simulink model "airgk"  (Simulink 3.00)
settings: Solver=ode45  StartTime=0  StopTime=Inf  RelTol=1e-3
libraries: simulink3 x21, airlib x1
(part 2 of 2)

== system airgk/uy-Control/uDynInv/Inertia Products ==
  w : Inport  Port=1  PortWidth=-1  SampleTime=-1  DataType=auto
      settings: SignalType=auto
  wd : Inport  Port=2  PortWidth=-1  SampleTime=-1  DataType=auto
      settings: SignalType=auto
  3x1mult : Subsystem
      mask Type: 3x1 Matrix Multiplication
      mask Description:
      | Input 1   : elements of matrix X (3 by 3)
      |   Input 2   : elements of matrix Y (3 by 1)
      |   Output   : elements of matrix X*Y (3 by 1)
      mask Help:
      | <p>
      | Elements of input and output matrices are taken columnwise.
      | </p>
      mask Display: disp('Z=X*Y')
  3x1mult1 : Subsystem
      mask Type: 3x1 Matrix Multiplication
      mask Description:
      | Input 1   : elements of matrix X (3 by 3)
      |   Input 2   : elements of matrix Y (3 by 1)
      |   Output   : elements of matrix X*Y (3 by 1)
      mask Help:
      | <p>
      | Elements of input and output matrices are taken columnwise.
      | </p>
      mask Display: disp('Z=X*Y')
  3x1mult2 : Subsystem
      mask Type: 3x1 Matrix Multiplication
      mask Description:
      | Input 1   : elements of matrix X (3 by 3)
      |   Input 2   : elements of matrix Y (3 by 1)
      |   Output   : elements of matrix X*Y (3 by 1)
      mask Help:
      | <p>
      | Elements of input and output matrices are taken columnwise.
      | </p>
      mask Display: disp('Z=X*Y')
  Inertia Matrix : Constant  Value=[GM1(4) -GM1(7) -GM1(8) -GM1(7) GM1(5) -GM1(9) -GM1(8) -GM1(9) GM1(6)]
  Sum : Sum  Inputs=|++  SaturateOnIntegerOverflow=on
  w2W : Subsystem
      mask Display: disp('S')
  W*J*w+J*wt : Outport  Port=1
  wires:
  w2W/1(Out1) -> 3x1mult2/1(X)
  3x1mult1/1(Z) -> 3x1mult2/2(Y)
  w/1 -> 3x1mult1/2(Y), w2W/1(In1)
  3x1mult/1(Z) -> Sum/1
  3x1mult2/1(Z) -> Sum/2
  Sum/1 -> W*J*w+J*wt/1
  wd/1 -> 3x1mult/2(Y)
  Inertia Matrix/1 -> 3x1mult/1(X), 3x1mult1/1(X)

== system airgk/uy-Control/uDynInv/Inv Rot ==
  w : Inport  Port=1  PortWidth=-1  SampleTime=-1  DataType=auto
      settings: SignalType=auto
  ftp : Inport  Port=2  PortWidth=-1  SampleTime=-1  DataType=auto
      settings: SignalType=auto
  add : Inport  Port=3  PortWidth=-1  SampleTime=-1  DataType=auto
      settings: SignalType=auto
  M : Subsystem
      mask Type: Simulink Matrix Library Block
      mask Description:
      | Roll, Pitch and Yaw derivatives to Omega :
      |   Input 1 : Roll, Pitch and Yaw angles (phi,theta,psi)
      |   Input 2 : Roll, Pitch and Yaw derivatives
      |   Output : Omega (p,q,r)
      mask Help:
      | <p>
      | Roll, Pitch and Yaw angles express the orientation
      | of the Body frame with respect to the Earth frame.
      | </p>
      | <p>
      | To use this block you should have the smxl library in your path.
      | </p>
  Sum1 : Sum  Inputs=+++  SaturateOnIntegerOverflow=on
  dM/df : Subsystem
  dM/dt : Subsystem
  pqr2ftpdot : Subsystem
      mask Type: Simulink Matrix Library Block
      mask Description:
      | Omega to Roll, Pitch and Yaw derivatives :
      |   Input 1 : Roll, Pitch and Yaw angles (phi,theta,psi)
      |   Input 2 : Omega (p,q,r)
      |   Output : Roll, Pitch and Yaw derivatives
      mask Help:
      | <p>
      | Roll, Pitch and Yaw angles express the orientation
      | of the Body frame with respect to the Earth frame.
      | </p>
      | <p>
      | To use this block you should have the smxl library in your path.
      | </p>
  wd : Outport  Port=1
  wires:
  add/1 -> M/2(ftpdot)
  ftp/1 -> pqr2ftpdot/1(ftp), M/1(ftp), dM/df/1(ftp), dM/dt/1(ftp)
  w/1 -> pqr2ftpdot/2(pqr)
  pqr2ftpdot/1(ftpdot) -> dM/dt/2(ftpd), dM/df/2(ftpd)
  M/1(pqr) -> Sum1/3
  dM/dt/1(Tt) -> Sum1/1
  dM/df/1(Tf) -> Sum1/2
  Sum1/1 -> wd/1

== system airgk/uy-Control/uDynInv/ad1 ==
  x : Inport  Port=1  PortWidth=-1  SampleTime=-1  DataType=auto
      settings: SignalType=auto
  yatm : Inport  Port=2  PortWidth=-1  SampleTime=-1  DataType=auto
      settings: SignalType=auto
  0 : Subsystem
      settings: OpenFcn=fdchelp airdata1
      mask Display: disp('AIRDATA1\nM.O. Rauw, October 1997')
  M : Fcn  Expr=u[2]/u[1]
  Mux : Mux  Inputs=[1 12]
      settings: DisplayOption=none
  Mux1 : Mux  Inputs=[12 5]
      settings: DisplayOption=none
  Mux2 : Mux  Inputs=3
      settings: DisplayOption=none
  a : Fcn  Expr=sqrt(401.8743*u[3])
  qdyn : Fcn  Expr=0.5*u[13]*u[1]^2
  yad1 : Outport  Port=1
  wires:
  yatm/1 -> Mux1/2, a/1
  x/1 -> Mux1/1, Mux/2
  Mux/1 -> M/1
  Mux1/1 -> qdyn/1
  M/1 -> Mux2/2
  a/1 -> Mux2/1, Mux/1
  qdyn/1 -> Mux2/3
  Mux2/1 -> yad1/1

== system airgk/uy-Control/uDynInv/atm ==
  x : Inport  Port=1  PortWidth=-1  SampleTime=-1  DataType=auto
      settings: SignalType=auto
  0 : Subsystem
      settings: OpenFcn=fdchelp atmosph
      mask Display: disp('ATMOSPH\nM.O. Rauw, October 1997')
  Mux : Mux  Inputs=2
      settings: DisplayOption=none
  Mux1 : Mux  Inputs=[2 1]
      settings: DisplayOption=none
  Mux2 : Mux  Inputs=5
      settings: DisplayOption=none
  T : Fcn  Expr=288.15 - 0.0065*u[12]
  g : Fcn  Expr=9.80665*(6371020/(6371020+u[12]))^2
  mu : Fcn  Expr=(1.458*10^(-6)*u[2]^1.5)/(u[2]+110.4)
  ps : Fcn  Expr=101325*(u[2]/288.15)^(u[1]/1.86584)
  rho : Fcn  Expr=u[3]/(287.053*u[2])
  yatm : Outport  Port=1
  wires:
  mu/1 -> Mux2/4
  Mux2/1 -> yatm/1
  Mux1/1 -> rho/1
  rho/1 -> Mux2/1
  g/1 -> Mux2/5, Mux/1
  T/1 -> Mux2/3, Mux/2
  ps/1 -> Mux2/2, Mux1/2
  Mux/1 -> ps/1, mu/1, Mux1/1
  x/1 -> g/1, T/1

== system airgk/uy-Control/uDynInv/dl ==
  x : Inport  Port=1  PortWidth=-1  SampleTime=-1  DataType=auto
      settings: SignalType=auto
  0 : Subsystem
      settings: OpenFcn=fdchelp dimless
      mask Display: disp('DIMLESS\nM.O. Rauw, October 1997')
  Mux : Mux  Inputs=3
      settings: DisplayOption=none
  pb/2V : Fcn  Expr=0.5 * u[4] * b / u[1]
  qc/2V : Fcn  Expr=0.5* u[5] * cbar / u[1]
  rb/2V : Fcn  Expr=0.5 * u[6] * b / u[1]
  ydl : Outport  Port=1
  wires:
  pb/2V/1 -> Mux/1
  qc/2V/1 -> Mux/2
  rb/2V/1 -> Mux/3
  Mux/1 -> ydl/1
  x/1 -> qc/2V/1, rb/2V/1, pb/2V/1

== system airgk/uy-Control/uDynInv/inv AM_CM ==
  In1 : Inport  Port=1  PortWidth=-1  SampleTime=-1  DataType=auto
      settings: SignalType=auto
  Matrix Gain : StateSpace  A=[]  B=[]  C=[]  D=M  X0=0
  Out1 : Outport  Port=1
  wires:
  In1/1 -> Matrix Gain/1
  Matrix Gain/1 -> Out1/1

== system airgk/uy-Control/4CmdsuKinInv/Exact Turn Coordination/Derivative ==
  x : Inport  Orientation=left  Port=1  PortWidth=-1  SampleTime=-1  DataType=auto
      settings: SignalType=auto
  Product2 : Product  Orientation=left  Inputs=/*  SaturateOnIntegerOverflow=on
  Sum4 : Sum  Orientation=left  Inputs=|+-  SaturateOnIntegerOverflow=on
  Unit Delay1 : UnitDelay  Orientation=left  X0=x0  SampleTime=T
  Zero-Order Hold1 : ZeroOrderHold  Orientation=left  SampleTime=T
  m : Constant  Orientation=left  Value=T
  xdot : Outport  Orientation=left  Port=1
  wires:
  Sum4/1 -> Product2/2
  Unit Delay1/1 -> Sum4/2
  Zero-Order Hold1/1 -> Sum4/1, Unit Delay1/1
  m/1 -> Product2/1
  Product2/1 -> xdot/1
  x/1 -> Zero-Order Hold1/1

== system airgk/uy-Control/4CmdsuKinInv/a2c  xy/Derivative ==
  x : Inport  Orientation=left  Port=1  PortWidth=-1  SampleTime=-1  DataType=auto
      settings: SignalType=auto
  Product2 : Product  Orientation=left  Inputs=/*  SaturateOnIntegerOverflow=on
  Sum4 : Sum  Orientation=left  Inputs=|+-  SaturateOnIntegerOverflow=on
  Unit Delay1 : UnitDelay  Orientation=left  X0=0  SampleTime=-1
  Zero-Order Hold1 : ZeroOrderHold  Orientation=left  SampleTime=T
  m : Constant  Orientation=left  Value=T
  xdot : Outport  Orientation=left  Port=1
  wires:
  x/1 -> Zero-Order Hold1/1
  Product2/1 -> xdot/1
  m/1 -> Product2/1
  Zero-Order Hold1/1 -> Unit Delay1/1, Sum4/1
  Unit Delay1/1 -> Sum4/2
  Sum4/1 -> Product2/2

== system airgk/uy-Control/4CmdsuKinInv/a2c xz/Derivative ==
  x : Inport  Orientation=left  Port=1  PortWidth=-1  SampleTime=-1  DataType=auto
      settings: SignalType=auto
  Product2 : Product  Orientation=left  Inputs=/*  SaturateOnIntegerOverflow=on
  Sum4 : Sum  Orientation=left  Inputs=|+-  SaturateOnIntegerOverflow=on
  Unit Delay1 : UnitDelay  Orientation=left  X0=0  SampleTime=-1
  Zero-Order Hold1 : ZeroOrderHold  Orientation=left  SampleTime=T
  m : Constant  Orientation=left  Value=T
  xdot : Outport  Orientation=left  Port=1
  wires:
  Sum4/1 -> Product2/2
  Unit Delay1/1 -> Sum4/2
  Zero-Order Hold1/1 -> Sum4/1, Unit Delay1/1
  m/1 -> Product2/1
  Product2/1 -> xdot/1
  x/1 -> Zero-Order Hold1/1

== system airgk/uy-Control/Vcmd Generator/xyHdot/3x1 ==
  X : Inport  Port=1  PortWidth=-1  SampleTime=-1  DataType=auto
      settings: SignalType=auto
  Y : Inport  Port=2  PortWidth=-1  SampleTime=-1  DataType=auto
      settings: SignalType=auto
  Dot Product1 : Subsystem  mask(Dot Product){}
      mask help:
      | Inner (dot) product.
      | y = sum(conj(u1).*u2). The operand u1 corresponds to the top (or left) input port.
      mask init:
      | t=(0:.1:2*pi)';
      | x=cos(t);
      | y=sin(t);
      | r=0.05;
      mask Help: Computes the inner (dot) product of the inputs: sum(u1.*u2).  The inputs are vectors of the same length. Output is a scalar.
      mask Display: patch([x*r+0.5],[y*r+0.5])
  Dot Product2 : Subsystem  mask(Dot Product){}
      mask help:
      | Inner (dot) product.
      | y = sum(conj(u1).*u2). The operand u1 corresponds to the top (or left) input port.
      mask init:
      | t=(0:.1:2*pi)';
      | x=cos(t);
      | y=sin(t);
      | r=0.05;
      mask Help: Computes the inner (dot) product of the inputs: sum(u1.*u2).  The inputs are vectors of the same length. Output is a scalar.
      mask Display: patch([x*r+0.5],[y*r+0.5])
  Dot Product9 : Subsystem  mask(Dot Product){}
      mask help:
      | Inner (dot) product.
      | y = sum(conj(u1).*u2). The operand u1 corresponds to the top (or left) input port.
      mask init:
      | t=(0:.1:2*pi)';
      | x=cos(t);
      | y=sin(t);
      | r=0.05;
      mask Help: Computes the inner (dot) product of the inputs: sum(u1.*u2).  The inputs are vectors of the same length. Output is a scalar.
      mask Display: patch([x*r+0.5],[y*r+0.5])
  Gain : Gain  Gain=-1  SaturateOnIntegerOverflow=off
  Mux : Mux  Inputs=3
  Selector : Selector  Elements=[1:3]  InputPortWidth=9
  Selector1 : Selector  Elements=[4:6]  InputPortWidth=9
  Selector2 : Selector  Elements=[7:9]  InputPortWidth=9
  Z : Outport  Port=1
  wires:
  Mux/1 -> Z/1
  Selector2/1 -> Dot Product2/1(In1)
  Selector1/1 -> Dot Product1/1(In1)
  Y/1 -> Dot Product9/2(In2), Dot Product1/2(In2), Dot Product2/2(In2)
  Dot Product2/1(Out1) -> Gain/1
  Dot Product1/1(Out1) -> Mux/2
  Dot Product9/1(Out1) -> Mux/1
  Selector/1 -> Dot Product9/1(In1)
  X/1 -> Selector2/1, Selector1/1, Selector/1
  Gain/1 -> Mux/3

== system airgk/uy-Control/Vcmd Generator/xyHdot/SinCos ==
  theta : Inport  Port=1  PortWidth=-1  SampleTime=-1  DataType=auto
      settings: SignalType=auto
  cosine : Trigonometry  Operator=cos  OutputSignalType=auto
  sine : Trigonometry  Operator=sin  OutputSignalType=auto
  sin(theta) : Outport  Port=1
  cos(theta) : Outport  Port=2
  wires:
  cosine/1 -> cos(theta)/1
  sine/1 -> sin(theta)/1
  theta/1 -> cosine/1, sine/1

== system airgk/uy-Control/uDynInv/ u term/uvw ==
  x : Inport  Port=1  PortWidth=-1  SampleTime=-1  DataType=auto
      settings: SignalType=auto
  Mux : Mux  Inputs=3
      settings: DisplayOption=none
  u : Fcn  Expr=u[1]*cos(u[2])*cos(u[3])
  v : Fcn  Expr=u[1]*sin(u[3])
  w : Fcn  Expr=u[1]*sin(u[2])*cos(u[3])
  ybvel : Outport  Port=1
  wires:
  Mux/1 -> ybvel/1
  w/1 -> Mux/3
  v/1 -> Mux/2
  u/1 -> Mux/1
  x/1 -> v/1, w/1, u/1

== system airgk/uy-Control/uDynInv/Inertia Products/3x1mult ==
  X : Inport  Port=1  PortWidth=-1  SampleTime=-1  DataType=auto
      settings: SignalType=auto
  Y : Inport  Port=2  PortWidth=-1  SampleTime=-1  DataType=auto
      settings: SignalType=auto
  Dot Product : simulink3/Math/Dot Product
  Dot Product1 : simulink3/Math/Dot Product
  Dot Product2 : simulink3/Math/Dot Product
  Mux : Mux  Inputs=3
  Selector : Selector  Elements=[0 3 6]+1  InputPortWidth=9
  Selector1 : Selector  Elements=[0 3 6]+2  InputPortWidth=9
  Selector2 : Selector  Elements=[0 3 6]+3  InputPortWidth=9
  Z : Outport  Port=1
  wires:
  Y/1 -> Dot Product/2, Dot Product1/2, Dot Product2/2
  Selector2/1 -> Dot Product2/1
  Selector1/1 -> Dot Product1/1
  Selector/1 -> Dot Product/1
  Mux/1 -> Z/1
  Dot Product2/1 -> Mux/3
  Dot Product1/1 -> Mux/2
  Dot Product/1 -> Mux/1
  X/1 -> Selector2/1, Selector1/1, Selector/1

== system airgk/uy-Control/uDynInv/Inertia Products/3x1mult1 ==
  X : Inport  Port=1  PortWidth=-1  SampleTime=-1  DataType=auto
      settings: SignalType=auto
  Y : Inport  Port=2  PortWidth=-1  SampleTime=-1  DataType=auto
      settings: SignalType=auto
  Dot Product : simulink3/Math/Dot Product
  Dot Product1 : simulink3/Math/Dot Product
  Dot Product2 : simulink3/Math/Dot Product
  Mux : Mux  Inputs=3
  Selector : Selector  Elements=[0 3 6]+1  InputPortWidth=9
  Selector1 : Selector  Elements=[0 3 6]+2  InputPortWidth=9
  Selector2 : Selector  Elements=[0 3 6]+3  InputPortWidth=9
  Z : Outport  Port=1
  wires:
  Y/1 -> Dot Product/2, Dot Product1/2, Dot Product2/2
  Selector2/1 -> Dot Product2/1
  Selector1/1 -> Dot Product1/1
  Selector/1 -> Dot Product/1
  Mux/1 -> Z/1
  Dot Product2/1 -> Mux/3
  Dot Product1/1 -> Mux/2
  Dot Product/1 -> Mux/1
  X/1 -> Selector2/1, Selector1/1, Selector/1

== system airgk/uy-Control/uDynInv/Inertia Products/3x1mult2 ==
  X : Inport  Port=1  PortWidth=-1  SampleTime=-1  DataType=auto
      settings: SignalType=auto
  Y : Inport  Port=2  PortWidth=-1  SampleTime=-1  DataType=auto
      settings: SignalType=auto
  Dot Product : simulink3/Math/Dot Product
  Dot Product1 : simulink3/Math/Dot Product
  Dot Product2 : simulink3/Math/Dot Product
  Mux : Mux  Inputs=3
  Selector : Selector  Elements=[0 3 6]+1  InputPortWidth=9
  Selector1 : Selector  Elements=[0 3 6]+2  InputPortWidth=9
  Selector2 : Selector  Elements=[0 3 6]+3  InputPortWidth=9
  Z : Outport  Port=1
  wires:
  Y/1 -> Dot Product/2, Dot Product1/2, Dot Product2/2
  Selector2/1 -> Dot Product2/1
  Selector1/1 -> Dot Product1/1
  Selector/1 -> Dot Product/1
  Mux/1 -> Z/1
  Dot Product2/1 -> Mux/3
  Dot Product1/1 -> Mux/2
  Dot Product/1 -> Mux/1
  X/1 -> Selector2/1, Selector1/1, Selector/1

== system airgk/uy-Control/uDynInv/Inertia Products/w2W ==
  In1 : Inport  Port=1  PortWidth=-1  SampleTime=-1  DataType=auto
      settings: SignalType=auto
  State Space : StateSpace  A=[]  B=[]  C=[]  D=[0 0 0;0 0 1;0 -1 0;0 0 -1;0 0 0;1 0 0;0 1 0;-1 0 0;0 0 0]  X0=0
  Out1 : Outport  Port=1
  wires:
  State Space/1 -> Out1/1
  In1/1 -> State Space/1

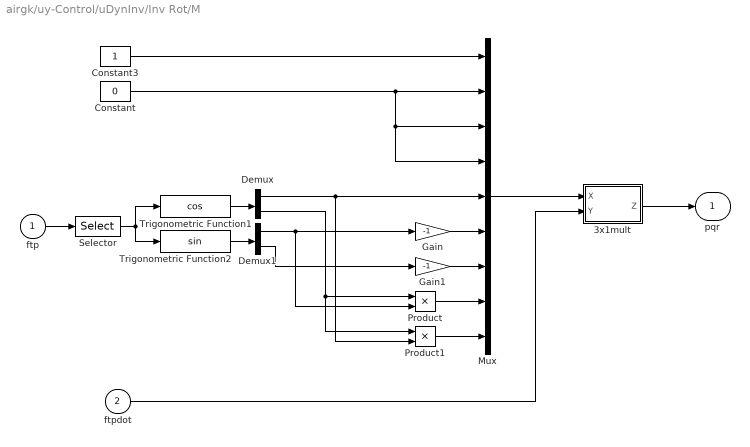
== system airgk/uy-Control/uDynInv/Inv Rot/M ==
  ftp : Inport  Port=1  PortWidth=-1  SampleTime=-1  DataType=auto
      settings: SignalType=auto
  ftpdot : Inport  Port=2  PortWidth=-1  SampleTime=-1  DataType=auto
      settings: SignalType=auto
  3x1mult : Subsystem
      mask Type: 3x1 Matrix Multiplication
      mask Description:
      | Input 1   : elements of matrix X (3 by 3)
      |   Input 2   : elements of matrix Y (3 by 1)
      |   Output   : elements of matrix X*Y (3 by 1)
      mask Help:
      | <p>
      | Elements of input and output matrices are taken columnwise.
      | </p>
      mask Display: disp('Z=X*Y')
  Constant : Constant  Value=0
  Constant3 : Constant  Value=1
  Demux : Demux  Outputs=2
  Demux1 : Demux  Outputs=2
  Gain : Gain  Gain=-1  SaturateOnIntegerOverflow=on
  Gain1 : Gain  Gain=-1  SaturateOnIntegerOverflow=on
  Mux : Mux  Inputs=9
  Product : Product  Inputs=2  SaturateOnIntegerOverflow=on
  Product1 : Product  Inputs=2  SaturateOnIntegerOverflow=on
  Selector : Selector  Elements=[1 2]  InputPortWidth=3
  Trigonometric Function1 : Trigonometry  Operator=cos  OutputSignalType=auto
  Trigonometric Function2 : Trigonometry  Operator=sin  OutputSignalType=auto
  pqr : Outport  Port=1
  wires:
  Constant3/1 -> Mux/1
  Constant/1 -> Mux/2, Mux/3, Mux/4
  Gain/1 -> Mux/6
  Gain1/1 -> Mux/7
  Trigonometric Function1/1 -> Demux/1
  Demux1/2 -> Gain1/1
  Product/1 -> Mux/8
  Product1/1 -> Mux/9
  Demux/2 -> Product/1, Product1/1
  Demux/1 -> Mux/5, Product1/2
  Selector/1 -> Trigonometric Function1/1, Trigonometric Function2/1
  ftpdot/1 -> 3x1mult/2(Y)
  Mux/1 -> 3x1mult/1(X)
  3x1mult/1(Z) -> pqr/1
  Trigonometric Function2/1 -> Demux1/1
  Demux1/1 -> Gain/1, Product/2
  ftp/1 -> Selector/1

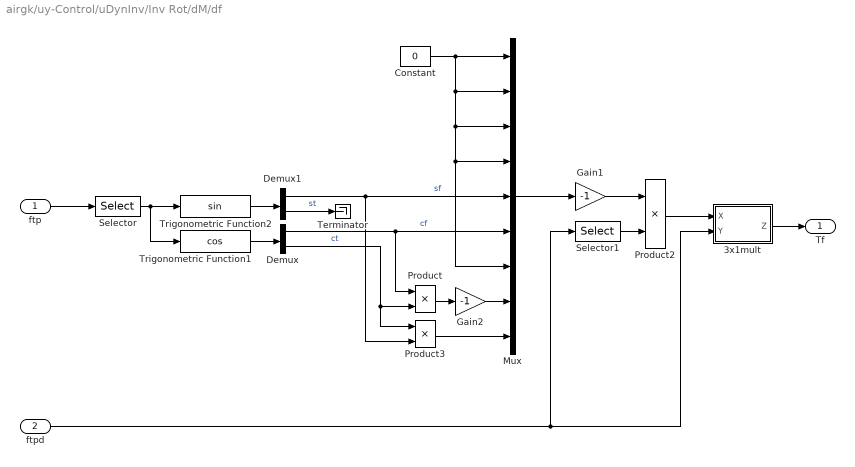
== system airgk/uy-Control/uDynInv/Inv Rot/dM/df ==
  ftp : Inport  Port=1  PortWidth=-1  SampleTime=-1  DataType=auto
      settings: SignalType=auto
  ftpd : Inport  Port=2  PortWidth=-1  SampleTime=-1  DataType=auto
      settings: SignalType=auto
  3x1mult : Subsystem
      mask Type: 3x1 Matrix Multiplication
      mask Description:
      | Input 1   : elements of matrix X (3 by 3)
      |   Input 2   : elements of matrix Y (3 by 1)
      |   Output   : elements of matrix X*Y (3 by 1)
      mask Help:
      | <p>
      | Elements of input and output matrices are taken columnwise.
      | </p>
      mask Display: disp('Z=X*Y')
  Constant : Constant  Value=0
  Demux : Demux  Outputs=2
  Demux1 : Demux  Outputs=2
  Gain1 : Gain  Gain=-1  SaturateOnIntegerOverflow=on
  Gain2 : Gain  Gain=-1  SaturateOnIntegerOverflow=on
  Mux : Mux  Inputs=9
  Product : Product  Inputs=2  SaturateOnIntegerOverflow=on
  Product2 : Product  Inputs=2  SaturateOnIntegerOverflow=on
  Product3 : Product  Inputs=2  SaturateOnIntegerOverflow=on
  Selector : Selector  Elements=[1 2]  InputPortWidth=3
  Selector1 : Selector  Elements=1  InputPortWidth=3
  Terminator : Terminator
  Trigonometric Function1 : Trigonometry  Operator=cos  OutputSignalType=auto
  Trigonometric Function2 : Trigonometry  Operator=sin  OutputSignalType=auto
  Tf : Outport  Port=1
  wires:
  3x1mult/1(Z) -> Tf/1
  Selector1/1 -> Product2/2
  Product2/1 -> 3x1mult/1(X)
  ftpd/1 -> Selector1/1, 3x1mult/2(Y)
  Gain1/1 -> Product2/1
  Mux/1 -> Gain1/1
  Constant/1 -> Mux/3, Mux/4, Mux/7, Mux/2, Mux/1
  ftp/1 -> Selector/1
  Trigonometric Function2/1 -> Demux1/1
  Selector/1 -> Trigonometric Function2/1, Trigonometric Function1/1
  Trigonometric Function1/1 -> Demux/1
  Demux1/1 -> Mux/5, Product3/2  "sf"
  Demux/1 -> Mux/6, Product/1  "cf"
  Product/1 -> Gain2/1
  Demux/2 -> Product/2, Product3/1  "ct"
  Product3/1 -> Mux/9
  Demux1/2 -> Terminator/1  "st"
  Gain2/1 -> Mux/8

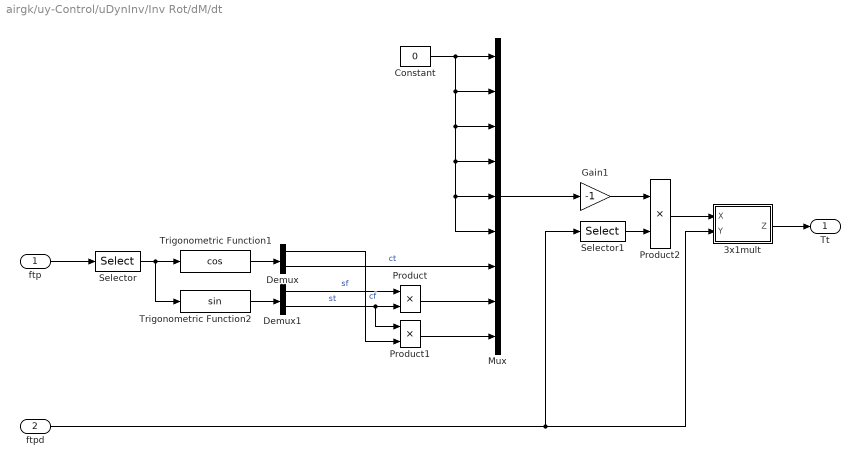
== system airgk/uy-Control/uDynInv/Inv Rot/dM/dt ==
  ftp : Inport  Port=1  PortWidth=-1  SampleTime=-1  DataType=auto
      settings: SignalType=auto
  ftpd : Inport  Port=2  PortWidth=-1  SampleTime=-1  DataType=auto
      settings: SignalType=auto
  3x1mult : Subsystem
      mask Type: 3x1 Matrix Multiplication
      mask Description:
      | Input 1   : elements of matrix X (3 by 3)
      |   Input 2   : elements of matrix Y (3 by 1)
      |   Output   : elements of matrix X*Y (3 by 1)
      mask Help:
      | <p>
      | Elements of input and output matrices are taken columnwise.
      | </p>
      mask Display: disp('Z=X*Y')
  Constant : Constant  Value=0
  Demux : Demux  Outputs=2
  Demux1 : Demux  Outputs=2
  Gain1 : Gain  Gain=-1  SaturateOnIntegerOverflow=on
  Mux : Mux  Inputs=9
  Product : Product  Inputs=2  SaturateOnIntegerOverflow=on
  Product1 : Product  Inputs=2  SaturateOnIntegerOverflow=on
  Product2 : Product  Inputs=2  SaturateOnIntegerOverflow=on
  Selector : Selector  Elements=[1 2]  InputPortWidth=3
  Selector1 : Selector  Elements=2  InputPortWidth=3
  Trigonometric Function1 : Trigonometry  Operator=cos  OutputSignalType=auto
  Trigonometric Function2 : Trigonometry  Operator=sin  OutputSignalType=auto
  Tt : Outport  Port=1
  wires:
  Trigonometric Function1/1 -> Demux/1
  Selector/1 -> Trigonometric Function2/1, Trigonometric Function1/1
  Trigonometric Function2/1 -> Demux1/1
  ftp/1 -> Selector/1
  Constant/1 -> Mux/1, Mux/2, Mux/3, Mux/4, Mux/5, Mux/6
  Demux/2 -> Mux/7  "ct"
  Product/1 -> Mux/8
  Product1/1 -> Mux/9
  Mux/1 -> Gain1/1
  Gain1/1 -> Product2/1
  Demux1/1 -> Product/1  "sf"
  Demux1/2 -> Product/2, Product1/1  "st"
  Demux/1 -> Product1/2  "cf"
  ftpd/1 -> 3x1mult/2(Y), Selector1/1
  Product2/1 -> 3x1mult/1(X)
  Selector1/1 -> Product2/2
  3x1mult/1(Z) -> Tt/1

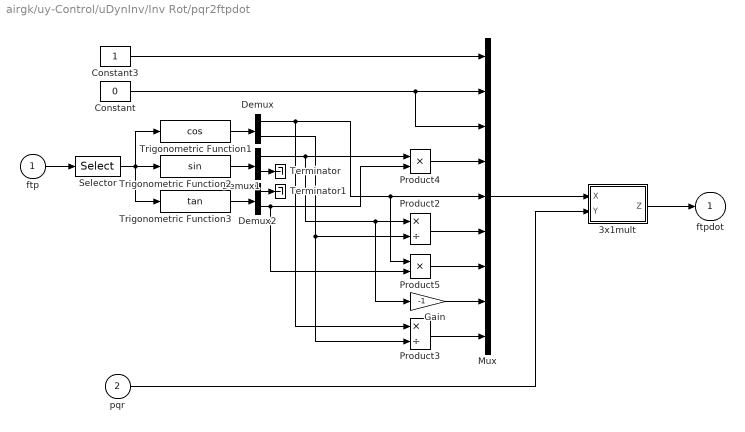
== system airgk/uy-Control/uDynInv/Inv Rot/pqr2ftpdot ==
  ftp : Inport  Port=1  PortWidth=-1  SampleTime=-1  DataType=auto
      settings: SignalType=auto
  pqr : Inport  Port=2  PortWidth=-1  SampleTime=-1  DataType=auto
      settings: SignalType=auto
  3x1mult : Subsystem
      mask Type: 3x1 Matrix Multiplication
      mask Description:
      | Input 1   : elements of matrix X (3 by 3)
      |   Input 2   : elements of matrix Y (3 by 1)
      |   Output   : elements of matrix X*Y (3 by 1)
      mask Help:
      | <p>
      | Elements of input and output matrices are taken columnwise.
      | </p>
      mask Display: disp('Z=X*Y')
  Constant : Constant  Value=0
  Constant3 : Constant  Value=1
  Demux : Demux  Outputs=2
  Demux1 : Demux  Outputs=2
  Demux2 : Demux  Outputs=2
  Gain : Gain  Gain=-1  SaturateOnIntegerOverflow=on
  Mux : Mux  Inputs=9
  Product2 : Product  Inputs=*/  SaturateOnIntegerOverflow=on
  Product3 : Product  Inputs=*/  SaturateOnIntegerOverflow=on
  Product4 : Product  Inputs=2  SaturateOnIntegerOverflow=on
  Product5 : Product  Inputs=2  SaturateOnIntegerOverflow=on
  Selector : Selector  Elements=[1 2]  InputPortWidth=3
  Terminator : Terminator
  Terminator1 : Terminator
  Trigonometric Function1 : Trigonometry  Operator=cos  OutputSignalType=auto
  Trigonometric Function2 : Trigonometry  Operator=sin  OutputSignalType=auto
  Trigonometric Function3 : Trigonometry  Operator=tan  OutputSignalType=auto
  ftpdot : Outport  Port=1
  wires:
  3x1mult/1(Z) -> ftpdot/1
  Mux/1 -> 3x1mult/1(X)
  pqr/1 -> 3x1mult/2(Y)
  Trigonometric Function3/1 -> Demux2/1
  Constant3/1 -> Mux/1
  Constant/1 -> Mux/2, Mux/3
  Product4/1 -> Mux/4
  Trigonometric Function2/1 -> Demux1/1
  Trigonometric Function1/1 -> Demux/1
  ftp/1 -> Selector/1
  Selector/1 -> Trigonometric Function2/1, Trigonometric Function3/1, Trigonometric Function1/1
  Demux1/1 -> Product4/1, Product2/1, Gain/1
  Product5/1 -> Mux/7
  Product2/1 -> Mux/6
  Demux2/2 -> Product4/2, Product5/2
  Demux/1 -> Mux/5, Product5/1, Product3/1
  Demux/2 -> Product2/2, Product3/2
  Product3/1 -> Mux/9
  Demux1/2 -> Terminator/1
  Demux2/1 -> Terminator1/1
  Gain/1 -> Mux/8

== system airgk/uy-Control/uDynInv/ad1/0 ==

== system airgk/uy-Control/uDynInv/atm/0 ==

== system airgk/uy-Control/uDynInv/dl/0 ==

== system airgk/uy-Control/Vcmd Generator/xyHdot/3x1/Dot Product1 ==
  In1 : Inport  Port=1  PortWidth=-1  SampleTime=-1  DataType=auto
      settings: SignalType=auto
  In2 : Inport  Port=2  PortWidth=-1  SampleTime=-1  DataType=auto
      settings: SignalType=auto
  S-Function : S-Function  FunctionName=sdotproduct  PortCounts=[]  SFunctionModules=''
  Out1 : Outport  Port=1
  wires:
  In2/1 -> S-Function/2
  In1/1 -> S-Function/1
  S-Function/1 -> Out1/1

== system airgk/uy-Control/Vcmd Generator/xyHdot/3x1/Dot Product2 ==
  In1 : Inport  Port=1  PortWidth=-1  SampleTime=-1  DataType=auto
      settings: SignalType=auto
  In2 : Inport  Port=2  PortWidth=-1  SampleTime=-1  DataType=auto
      settings: SignalType=auto
  S-Function : S-Function  FunctionName=sdotproduct  PortCounts=[]  SFunctionModules=''
  Out1 : Outport  Port=1
  wires:
  S-Function/1 -> Out1/1
  In1/1 -> S-Function/1
  In2/1 -> S-Function/2

== system airgk/uy-Control/Vcmd Generator/xyHdot/3x1/Dot Product9 ==
  In1 : Inport  Port=1  PortWidth=-1  SampleTime=-1  DataType=auto
      settings: SignalType=auto
  In2 : Inport  Port=2  PortWidth=-1  SampleTime=-1  DataType=auto
      settings: SignalType=auto
  S-Function : S-Function  FunctionName=sdotproduct  PortCounts=[]  SFunctionModules=''
  Out1 : Outport  Port=1
  wires:
  S-Function/1 -> Out1/1
  In1/1 -> S-Function/1
  In2/1 -> S-Function/2

== system airgk/uy-Control/uDynInv/Inv Rot/M/3x1mult ==
  X : Inport  Port=1  PortWidth=-1  SampleTime=-1  DataType=auto
      settings: SignalType=auto
  Y : Inport  Port=2  PortWidth=-1  SampleTime=-1  DataType=auto
      settings: SignalType=auto
  Dot Product : simulink3/Math/Dot Product
  Dot Product1 : simulink3/Math/Dot Product
  Dot Product2 : simulink3/Math/Dot Product
  Mux : Mux  Inputs=3
  Selector : Selector  Elements=[0 3 6]+1  InputPortWidth=9
  Selector1 : Selector  Elements=[0 3 6]+2  InputPortWidth=9
  Selector2 : Selector  Elements=[0 3 6]+3  InputPortWidth=9
  Z : Outport  Port=1
  wires:
  Y/1 -> Dot Product/2, Dot Product1/2, Dot Product2/2
  Selector2/1 -> Dot Product2/1
  Selector1/1 -> Dot Product1/1
  Selector/1 -> Dot Product/1
  Mux/1 -> Z/1
  Dot Product2/1 -> Mux/3
  Dot Product1/1 -> Mux/2
  Dot Product/1 -> Mux/1
  X/1 -> Selector2/1, Selector1/1, Selector/1

== system airgk/uy-Control/uDynInv/Inv Rot/dM/df/3x1mult ==
  X : Inport  Port=1  PortWidth=-1  SampleTime=-1  DataType=auto
      settings: SignalType=auto
  Y : Inport  Port=2  PortWidth=-1  SampleTime=-1  DataType=auto
      settings: SignalType=auto
  Dot Product : simulink3/Math/Dot Product
  Dot Product1 : simulink3/Math/Dot Product
  Dot Product2 : simulink3/Math/Dot Product
  Mux : Mux  Inputs=3
  Selector : Selector  Elements=[0 3 6]+1  InputPortWidth=9
  Selector1 : Selector  Elements=[0 3 6]+2  InputPortWidth=9
  Selector2 : Selector  Elements=[0 3 6]+3  InputPortWidth=9
  Z : Outport  Port=1
  wires:
  Y/1 -> Dot Product/2, Dot Product1/2, Dot Product2/2
  Selector2/1 -> Dot Product2/1
  Selector1/1 -> Dot Product1/1
  Selector/1 -> Dot Product/1
  Mux/1 -> Z/1
  Dot Product2/1 -> Mux/3
  Dot Product1/1 -> Mux/2
  Dot Product/1 -> Mux/1
  X/1 -> Selector2/1, Selector1/1, Selector/1

== system airgk/uy-Control/uDynInv/Inv Rot/dM/dt/3x1mult ==
  X : Inport  Port=1  PortWidth=-1  SampleTime=-1  DataType=auto
      settings: SignalType=auto
  Y : Inport  Port=2  PortWidth=-1  SampleTime=-1  DataType=auto
      settings: SignalType=auto
  Dot Product : simulink3/Math/Dot Product
  Dot Product1 : simulink3/Math/Dot Product
  Dot Product2 : simulink3/Math/Dot Product
  Mux : Mux  Inputs=3
  Selector : Selector  Elements=[0 3 6]+1  InputPortWidth=9
  Selector1 : Selector  Elements=[0 3 6]+2  InputPortWidth=9
  Selector2 : Selector  Elements=[0 3 6]+3  InputPortWidth=9
  Z : Outport  Port=1
  wires:
  Y/1 -> Dot Product/2, Dot Product1/2, Dot Product2/2
  Selector2/1 -> Dot Product2/1
  Selector1/1 -> Dot Product1/1
  Selector/1 -> Dot Product/1
  Mux/1 -> Z/1
  Dot Product2/1 -> Mux/3
  Dot Product1/1 -> Mux/2
  Dot Product/1 -> Mux/1
  X/1 -> Selector2/1, Selector1/1, Selector/1

== system airgk/uy-Control/uDynInv/Inv Rot/pqr2ftpdot/3x1mult ==
  X : Inport  Port=1  PortWidth=-1  SampleTime=-1  DataType=auto
      settings: SignalType=auto
  Y : Inport  Port=2  PortWidth=-1  SampleTime=-1  DataType=auto
      settings: SignalType=auto
  Dot Product : simulink3/Math/Dot Product
  Dot Product1 : simulink3/Math/Dot Product
  Dot Product2 : simulink3/Math/Dot Product
  Mux : Mux  Inputs=3
  Selector : Selector  Elements=[0 3 6]+1  InputPortWidth=9
  Selector1 : Selector  Elements=[0 3 6]+2  InputPortWidth=9
  Selector2 : Selector  Elements=[0 3 6]+3  InputPortWidth=9
  Z : Outport  Port=1
  wires:
  Y/1 -> Dot Product/2, Dot Product1/2, Dot Product2/2
  Selector2/1 -> Dot Product2/1
  Selector1/1 -> Dot Product1/1
  Selector/1 -> Dot Product/1
  Mux/1 -> Z/1
  Dot Product2/1 -> Mux/3
  Dot Product1/1 -> Mux/2
  Dot Product/1 -> Mux/1
  X/1 -> Selector2/1, Selector1/1, Selector/1
